simulink model "basicOpenLoopMSD"  (R2021a)
settings: Solver=FixedStepAuto  StartTime=0.0  StopTime=10  FixedStep=0.001  RelTol=1e-3
model workspace (MAT data in the model file):
  b = Simulink.Parameter
  b.Value = 1
  b.DataType = 'int8'
  b.Dimensions = [1 1]
  k = Simulink.Parameter
  k.Value = 4
  k.DataType = 'int8'
  k.Dimensions = [1 1]
  m = Simulink.Parameter
  m.Value = 1
  m.DataType = 'int8'
  m.Dimensions = [1 1]
undefined symbols (not defined in the file): DiscIntNeverNeededParam
settings Model: OrderedModelArguments=off  Creator=User  LastModifiedBy=User
settings DataIOCC: SaveOutput=off  SaveTime=off
settings OptimizationCC: DefaultParameterBehavior=Inlined  EnhancedBackFolding=on  PassReuseOutputArgsAs=Individual arguments  ZeroExternalMemoryAtStartup=off  ZeroInternalMemoryAtStartup=off  OptimizeBlockOrder=speed  DifferentSizesBufferReuse=on  OptimizationCustomize=off  EfficientTunableParamExpr=on
settings DebuggingCC: ParameterTunabilityLossMsg=error
settings SFSimCC: MATLABDynamicMemAlloc=off
settings RTWCC: SystemTargetFile=ert.tlc  TemplateMakefile=ert_default_tmf
settings CodeAppCC: ForceParamTrailComments=on  IgnoreCustomStorageClasses=off  OperatorAnnotations=on  SimulinkDataObjDesc=on  SFDataObjDesc=on  InsertBlockDesc=on
settings ERTTargetCC: TargetLangStandard=C99 (ISO)  GenerateSampleERTMain=on  SupportContinuousTime=on  InlinedParameterPlacement=NonHierarchical  ERTCustomFileTemplate=example_file_process.tlc
settings ConfigComp: CovEnable=on  CovScope=ReferencedModels  CovIncludeTopModel=off  CovMetricSettings=dcmwe  CovModelRefEnable=filtered

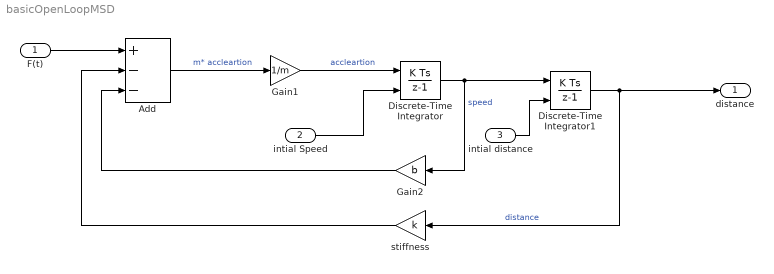
== system basicOpenLoopMSD ==
  F(t) : Inport  OutDataTypeStr=double  PortDimensions=1
  intial Speed : Inport  Port=2  OutDataTypeStr=double  PortDimensions=1
  intial distance : Inport  Port=3  OutDataTypeStr=double  PortDimensions=1
  Add : Sum  Inputs=+--
  Discrete-Time Integrator : DiscreteIntegrator  InitialConditionSource=external  SampleTime=-1  ICPrevOutput=DiscIntNeverNeededParam  ICPrevScaledInput=DiscIntNeverNeededParam
  Discrete-Time Integrator1 : DiscreteIntegrator  InitialConditionSource=external  SampleTime=-1  ICPrevOutput=DiscIntNeverNeededParam  ICPrevScaledInput=DiscIntNeverNeededParam
  Gain1 : Gain  Gain=1/m
  Gain2 : Gain  Gain=b
  stiffness : Gain  Gain=k
  distance : Outport  OutDataTypeStr=double  PortDimensions=1  SampleTime=0
  wires:
  intial Speed/1 -> Discrete-Time Integrator/2
  Discrete-Time Integrator/1 -> Discrete-Time Integrator1/1, Gain2/1  "speed"
  Gain1/1 -> Discrete-Time Integrator/1  "accleartion"
  intial distance/1 -> Discrete-Time Integrator1/2
  Add/1 -> Gain1/1  "m* accleartion"
  Gain2/1 -> Add/3
  stiffness/1 -> Add/2
  Discrete-Time Integrator1/1 -> stiffness/1, distance/1  "distance"
  F(t)/1 -> Add/1
